simulink model "Frdm_KL25Z"  (R2016b)
settings: Solver=FixedStepDiscrete  StartTime=0.0  StopTime=10.0  RelTol=1e-3  EnableMultiTasking=on
libraries: frdmtfcshieldlib x6, frdmkl25zlib x1
settings Model: ExtModeTrigDuration=5  Creator=jays  LastModifiedBy=VasutornSIRIYAKORN
settings OptimizationCC: MaxStackSize=64
settings DebuggingCC: ParameterTunabilityLossMsg=error
settings HardwareCC: ProdBitPerPointer=32  ProdBitPerSizeT=32  ProdBitPerPtrDiffT=32  ProdLargestAtomicInteger=Long  ProdLargestAtomicFloat=Double  ProdWordSize=32  ProdHWDeviceType=ARM Compatible->ARM Cortex
settings RTWCC: SystemTargetFile=ert.tlc  HardwareBoard=NXP FRDM-KL25Z  TLCOptions=-aInlineSetEventsForThisBaseRateFcn=TLC_FALSE -aSuppressMultiTaskScheduler=TLC_FALSE -aRateBasedStepFcn=1  TemplateMakefile=ert_default_tmf  Description=Embedded Coder  GenerateReport=on  Toolchain=GNU Tools for ARM Embedded Processors  IncludeHyperlinkInReport=on  LaunchReport=on  GenerateTraceInfo=on  GenerateTraceReport=on  GenerateTraceReportSl=on  GenerateTraceReportSf=on  GenerateTraceReportEml=on
settings CodeAppCC: ForceParamTrailComments=on  IgnoreCustomStorageClasses=off  OperatorAnnotations=on  SimulinkDataObjDesc=on  SFDataObjDesc=on  MATLABFcnDesc=on  InsertBlockDesc=on  MATLABSourceComments=on

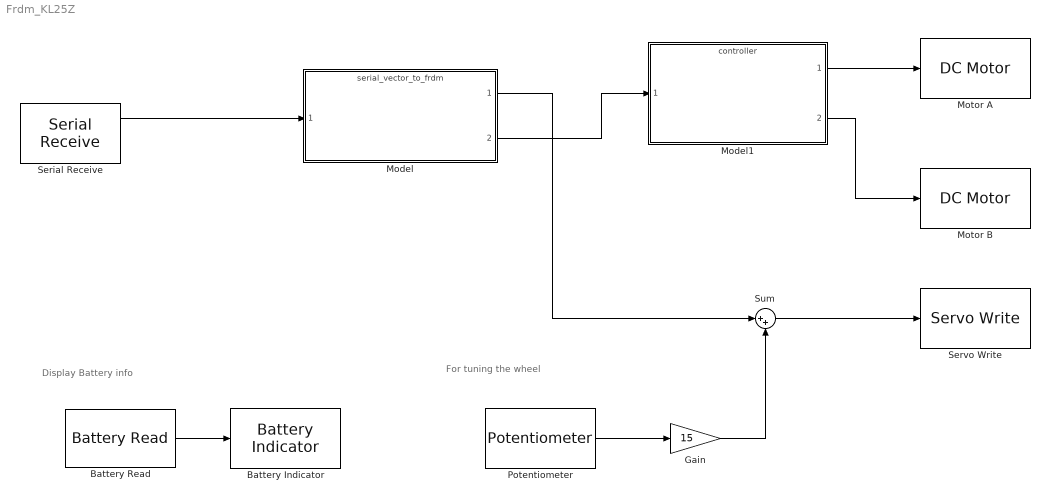
== system Frdm_KL25Z ==
  note: Display Battery info
  note: For tuning the wheel
  Battery Indicator : frdmtfcshieldlib/Battery Indicator
  Battery Read : frdmtfcshieldlib/Battery Read  SampleTime=0.01
  Gain : Gain  Gain=15
  Model : ModelReference  ModelNameDialog=serial_vector_to_frdm.slx  SimulationMode=Normal  ModelReferenceVersion=1.10
  Model1 : ModelReference  ModelNameDialog=controller.slx  SimulationMode=Normal  ModelReferenceVersion=1.7
  Motor A : frdmtfcshieldlib/DC Motor  WhichMotor=A
  Motor B : frdmtfcshieldlib/DC Motor  WhichMotor=B
  Potentiometer : frdmtfcshieldlib/Potentiometer  WhichPot=A  SampleTime=0.01
  Serial Receive : frdmkl25zlib/Serial Receive  uart=UART0  DataType=int8  DataLength=2  SampleTime=0.01
  Servo Write : frdmtfcshieldlib/Servo Write  WhichServo=0  minAngle=-35  maxAngle=35
  Sum : Sum  Inputs=|++
  wires:
  Model/1 -> Sum/1
  Battery Read/1 -> Battery Indicator/1
  Serial Receive/1 -> Model/1
  Model1/1 -> Motor A/1
  Model1/2 -> Motor B/1
  Potentiometer/1 -> Gain/1
  Gain/1 -> Sum/2
  Sum/1 -> Servo Write/1
  Model/2 -> Model1/1
